simulink model "BatteryStateOfCharge"  (R2016b)
settings: Solver=VariableStepAuto  StartTime=0.0  StopTime=sim_time  RelTol=1e-3
values from neighbouring files (symbols this model uses):
  Cn = 2.3 *3600    (= 8280)    [Battery_SOC_OCV_Management.m]
  I = 2.3    [Battery_SOC_OCV_Management.m]
  OCV = Data(:,2)    [Battery_SOC_OCV_Management.m]
  R_Charge = Data(:,3)    [Battery_SOC_OCV_Management.m]
  R_Discharge = Data(:,4)    [Battery_SOC_OCV_Management.m]
  SOC = Data(:,1)    [Battery_SOC_OCV_Management.m]
settings Model: Creator=1026691  LastModifiedBy=1026691

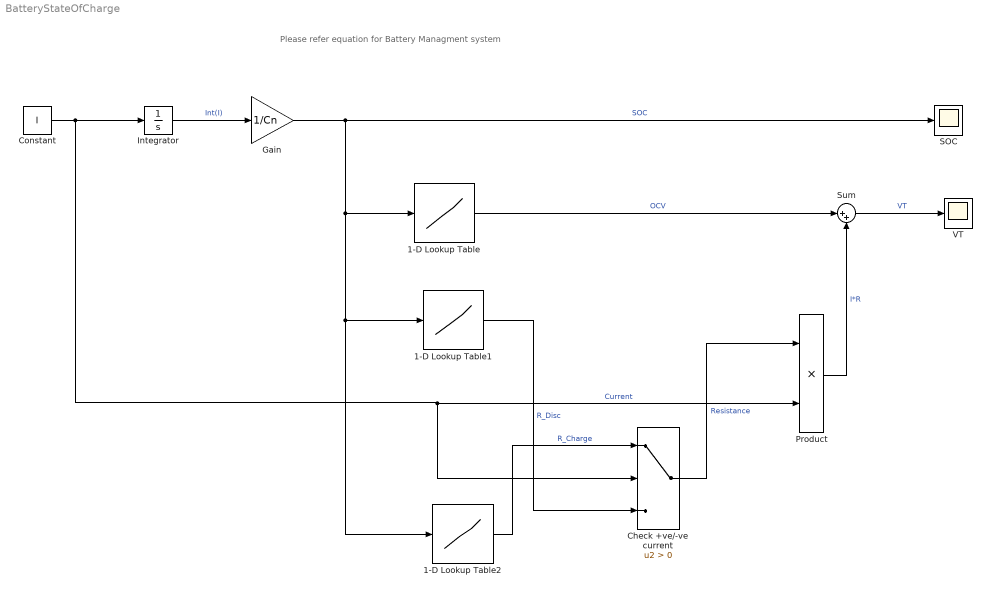
== system BatteryStateOfCharge ==
  note: Please refer equation for Battery Managment system
  1-D Lookup Table : Lookup_n-D  NumberOfTableDimensions=1  BreakpointsForDimension1=SOC  Table=OCV  InternalRulePriority=Speed  RndMeth=Simplest  InputSameDT=on
  1-D Lookup Table1 : Lookup_n-D  NumberOfTableDimensions=1  BreakpointsForDimension1=SOC  Table=R_Discharge  InternalRulePriority=Speed  RndMeth=Simplest  InputSameDT=on
  1-D Lookup Table2 : Lookup_n-D  NumberOfTableDimensions=1  BreakpointsForDimension1=SOC  Table=R_Charge  InternalRulePriority=Speed  RndMeth=Simplest  InputSameDT=on
  "Check +ve/-ve current " : Switch  Criteria=u2 > Threshold
  Constant : Constant  Value=I
  Gain : Gain  Gain=1/Cn
  Integrator : Integrator
  Product : Product
  SOC : Scope
  Sum : Sum  Inputs=|++
  VT : Scope
  wires:
  Constant/1 -> "Check +ve/-ve current "/2, Product/2, Integrator/1  "Current"
  Integrator/1 -> Gain/1  "Int(I)"
  Gain/1 -> SOC/1, 1-D Lookup Table2/1, 1-D Lookup Table1/1, 1-D Lookup Table/1  "SOC"
  1-D Lookup Table/1 -> Sum/1  "OCV"
  Product/1 -> Sum/2  "I*R"
  Sum/1 -> VT/1  "VT"
  1-D Lookup Table1/1 -> "Check +ve/-ve current "/3  "R_Disc"
  1-D Lookup Table2/1 -> "Check +ve/-ve current "/1  "R_Charge"
  "Check +ve/-ve current "/1 -> Product/1  "Resistance"
